simulink model "fenglijimoxing"  (R2014a)
settings: Solver=ode45  StartTime=0.0  StopTime=10.0  RelTol=1e-3
settings Model: Creator=hsinwang  LastModifiedBy=hsinwang

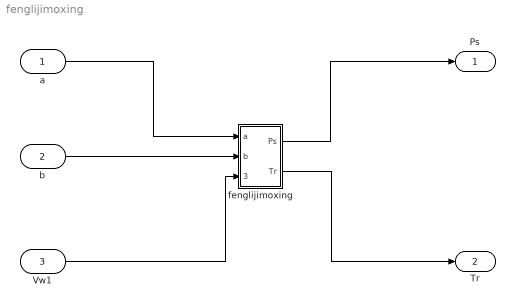
== system fenglijimoxing ==
  "a " : Inport
  b : Inport  Port=2
  Vw1 : Inport  Port=3
  "fenglijimoxing " : Subsystem
  " Ps " : Outport
  " Tr " : Outport  Port=2
  wires:
  b/1 -> "fenglijimoxing "/2(b)
  Vw1/1 -> "fenglijimoxing "/3(Vw1)
  "fenglijimoxing "/1("Ps ") -> " Ps "/1
  "fenglijimoxing "/2(" Tr ") -> " Tr "/1
  "a "/1 -> "fenglijimoxing "/1("a ")

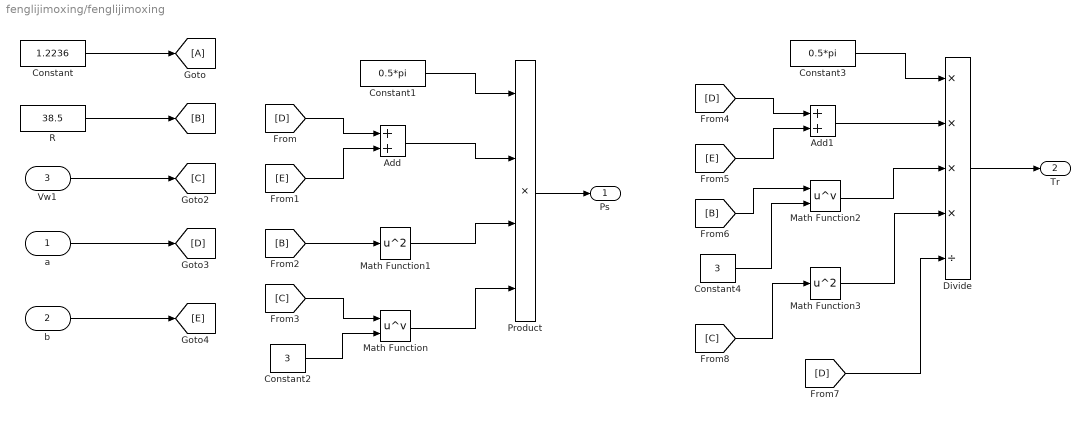
== system fenglijimoxing/fenglijimoxing  ==
  "a " : Inport
  b : Inport  Port=2
  Vw1 : Inport  Port=3
  Add : Sum
  Add1 : Sum
  Constant : Constant  Value=1.2236
  Constant1 : Constant  Value=0.5*pi
  Constant2 : Constant  Value=3
  Constant3 : Constant  Value=0.5*pi
  Constant4 : Constant  Value=3
  Divide : Product  Inputs=****/
  Math Function : Math  Operator=pow  SaturateOnIntegerOverflow=on
  Math Function1 : Math  Operator=square  SaturateOnIntegerOverflow=on
  Math Function2 : Math  Operator=pow  SaturateOnIntegerOverflow=on
  Math Function3 : Math  Operator=square  SaturateOnIntegerOverflow=on
  Product : Product  Inputs=4
  R : Constant  Value=38.5
  "Ps " : Outport
  " Tr " : Outport  Port=2
  wires:
  Math Function2/1 -> Divide/3
  Math Function1/1 -> Product/3
  Product/1 -> "Ps "/1
  [C] -> Math Function3/1
  Add/1 -> Product/2
  [D] -> Add/1
  [D] -> Divide/5
  Math Function3/1 -> Divide/4
  [B] -> Math Function2/1
  [D] -> Add1/1
  Constant4/1 -> Math Function2/2
  [E] -> Add/2
  Math Function/1 -> Product/4
  [E] -> Add1/2
  Constant3/1 -> Divide/1
  Divide/1 -> " Tr "/1
  Add1/1 -> Divide/2
  Constant/1 -> [A]
  Vw1/1 -> [C]
  b/1 -> [E]
  R/1 -> [B]
  "a "/1 -> [D]
  [C] -> Math Function/1
  Constant2/1 -> Math Function/2
  [B] -> Math Function1/1
  Constant1/1 -> Product/1
